simulink model "GridConnected200921_DSMC_OK_2018"  (R2022b)
settings: Solver=ode45  StartTime=0.0  StopTime=1  RelTol=1e-3
InitFcn:
  | %tham so mach nghich luu nguon ap mot pha
  | Li = 0.423e-3+0.429e-3;
  | rLi = 0.172+0.167;
  | Lg = 0.795e-3;
  | rLg = 0.36;
  | 
  | Lf = 0.8*(Li+Lg);
  | rL = (rLi+rLg);
  | 
  | Cdc = 0.9*2*470e-6;
  | P = 2500;  %Cong suat 2.5kW
  | VdcRated = 400; %Dien ap dat 400VDC
  | Rmin = (VdcRated^2)/P; %Full load
  | Rmax = (VdcRated^2)/(0.05*P); % 5% load
  | Fs = 10000;
  | Ts = 1/Fs;
StopFcn:
  | figure(1);
  | subplot(2,1,1); hold on; grid on;
  | plot(Vdc_Ref.time, Vdc_Ref.signals.values,'-k','Linewidth',1.5);
  | plot(Vdc_Fb.time, Vdc_Fb.signals.values,'r','Linewidth',1.5);
  | plot(Vdc_Filter.time, Vdc_Filter.signals.values,'b','Linewidth',1.5);
  | legend('Vdc Ref','Vdc Fb','Vdc Filter');
  | xlabel('Time(s)'); ylabel('Dc bus voltage(V)');
  | 
  | subplot(2,1,2); hold on; grid on;
  | [hAx,hLine1,hLine2] = plotyy(P.time, P.signals.values./1000, Q.time, Q.signals.values./1000);
  | set(hAx(1),'YLim',[-10 10]);
  | set(hAx(2),'YLim',[-10 10]);
  | set(hAx(1),'YTick',[-10:5:10]);
  | set(hAx(2),'YTick',[-10:5:10]);
  | ylabel(hAx(1),'P(kW)'); ylabel(hAx(2),'Q(kVar)');
  | legend('Active power','Reactive power');
  | set(hAx(1),'Fontsize',20);
  | set(hAx(2),'Fontsize',20)
  | xlabel('Time(s)'); ylabel('Injected power');
  | 
  | figure(2);
  | hold on; grid on;
  | plot(iL_Ref.time, iL_Ref.signals.values,'-.g','Linewidth',1.5);
  | plot(iL_avg.time, iL_avg.signals.values,'r','Linewidth',1.5);
  | plot(iL.time, iL.signals.values,'b','Linewidth',1.5);
  | legend('iL Ref','iL average','iL');
  | xlabel('Time(s)'); ylabel('Output current(A)');
  | %magnifyOnFigure();
  | 
  | figure(3);
  | subplot(2,1,1); hold on; grid on;
  | [hAx,hLine1,hLine2] = plotyy(V_Line.time, V_Line.signals.values, iL.time, iL.signals.values);
  | set(hAx(1),'YLim',[-400 400]);
  | set(hAx(2),'YLim',[-60 60]);
  | set(hAx(1),'YTick',[-400:200:400]);
  | set(hAx(2),'YTick',[-60:30:60]);
  | ylabel(hAx(1),'Line voltage(V)'); ylabel(hAx(2),'Injected current(A)');
  | legend('Line voltage','Injected current');
  | set(hAx(1),'Fontsize',20);
  | set(hAx(2),'Fontsize',20)
  | xlabel('Time(s)');
  | 
  | subplot(2,1,2);  hold on; grid on;
  | plot(Vdc_Ref.time, Vdc_Ref.signals.values,'-k','Linewidth',1.5);
  | plot(Vdc_Fb.time, Vdc_Fb.signals.values,'r','Linewidth',1.5);
  | plot(Vdc_Filter.time, Vdc_Filter.signals.values,'b','Linewidth',1.5);
  | legend('Vdc Ref','Vdc Fb','Vdc Filter');
  | xlabel('Time(s)'); ylabel('Dc bus voltage(V)');
  | %magnifyOnFigure();
  | 
  | figure(4);
  | subplot(2,1,1); hold on; grid on;
  | plot(V_Line.time, V_Line.signals.values,'r','Linewidth',1.5);
  | subplot(2,1,2); hold on; grid on;
  | plot(Theta.time, Theta.signals.values,'b','Linewidth',1.5);
  | 
  | figure(5);
  | subplot(2,1,1); hold on; grid on;
  | plot(V_Line.time, V_Line.signals.values,'r','Linewidth',1.5);
  | xlabel('Time(s)'); ylabel('Line voltage(V)');
  | subplot(2,1,2); hold on; grid on;
  | plot(iL.time, iL.signals.values,'b','Linewidth',1.5);
  | xlabel('Time(s)'); ylabel('Injected current(A)');
undefined symbols (not defined in the file): Vdc
libraries: spsSeriesRLCBranchLib x7, spsVoltageMeasurementLib x5, spsIGBTLib x4, spsIGBTDiodeLib x4, spsBreakerLib x3, spsCurrentMeasurementLib x2, spsControlledVoltageSourceLib x1, spsControlledCurrentSourceLib x1, spsTriangleGeneratorLib x1, spspowerguiLib x1
settings Model: Creator=ADMIN  LastModifiedBy=Dell
settings SolverCC: AlgebraicLoopSolver=TrustRegion
settings DataIOCC: ReturnWorkspaceOutputs=off
settings DebuggingCC: UnconnectedInputMsg=warning  UnconnectedOutputMsg=warning  UnconnectedLineMsg=warning  SFMachineParentedDataDiag=warning  ArithmeticOperatorsInVariantConditions=warning
settings ModelReferenceCC: EnableRefExpFcnMdlSchedulingChecks=on
settings SFSimCC: SimUseLocalCustomCode=off  CustomCodeUndefinedFunction=UseInterfaceOnly
settings RTWCC: RTWUseLocalCustomCode=off

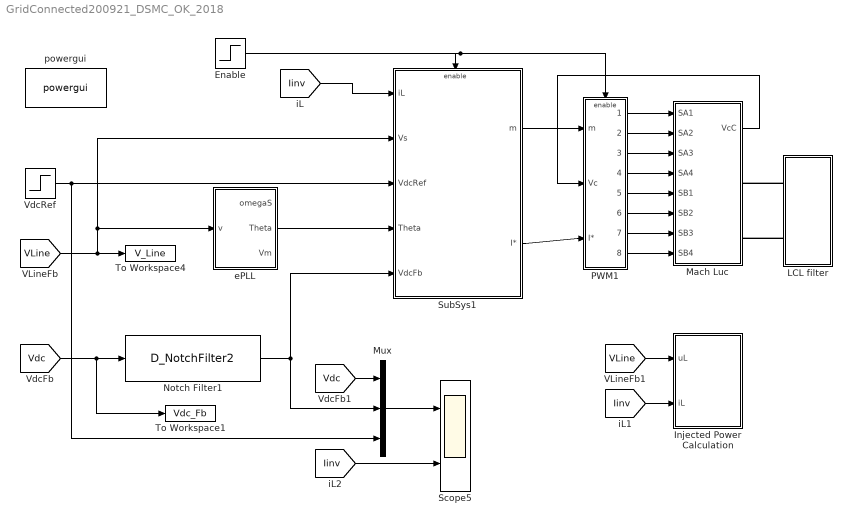
== system GridConnected200921_DSMC_OK_2018 ==
  Enable : Step  Time=0.1  SampleTime=0
  Injected Power Calculation : Subsystem
  LCL filter : Subsystem
  Mach Luc : Subsystem
  Mux : Mux  Inputs=3
  Notch Filter1 : S-Function  InitFcn=try, set_param(gcb,'FunctionName','D_NotchFilter2'), end  FunctionName=D_NotchFilter2  SFunctionModules=D_NotchFilter2_wrapper  SFunctionDeploymentMode=off  EnableBusSupport=off  mask(S-Function Builder){}
      mask help: Simulink:masks:SFunctionBuilder_MD
      mask init:
      | val = [[.9  0.75 0.75 1 1 .9 .9 1]',[1 1 0.75 0.75 .9 .9 1 .9]'];try , sys = get_param(gcb,'SfunBuilderFcnName');if isempty(sys), sys = get_param(gcb,'FunctionName'); end,catch, sys = get_param(gcb,'FunctionName'); end
      settings: CopyFcn=set_param(gcbh,'LinkStatus','none')  PreSaveFcn=try, set_param(gcb,'FunctionName','D_NotchFilter2'), end  OpenFcn=sfunctionwizard(gcbh)
      mask Display: plot(val(:,1),val(:,2)),disp(sys), port_label('input',1,'uDC'), port_label('output',1,'uDCav')
  PWM1 : Subsystem
  Scope5 : Scope  NumInputPorts=2
  SubSys1 : Subsystem
  To Workspace1 : ToWorkspace  VariableName=Vdc_Fb  SaveFormat=Structure With Time  SampleTime=1e-4
  To Workspace4 : ToWorkspace  VariableName=V_Line  SaveFormat=Structure With Time  SampleTime=1e-4
  VdcRef : Step  Time=0  After=400  SampleTime=0
  ePLL : Subsystem
  powergui : spspowerguiLib/powergui  Priority=1  SimulationMode=Discrete  SampleTime=5e-8  frequency=60  Iterations=50  frequencyindice=0  Pbase=100e6  ErrMax=1e-4  UnitsV=kV  UnitsW=MW  buscounter=0  FunctionMessages=off  echomessages=off  EnableUseOfTLC=off  CurrentSourceSwitches=off  DisableSnubberDevices=off  DisableRonSwitches=off  DisableVfSwitches=off  DisplayEquations=off  AutomaticDiscreteSolvers=off  SolverType=Tustin/Backward Euler (TBE)  Interpol=off  ExternalGateDelay=off  methode=off  Ts=100  x0status=blocks  SPID=off  SwTol=0  HookPort=off  NonlinearTolerance=1e-4  nMaxIteration=100  ContinueOnMaxIteration=off  RestoreLinks=warning  ResistiveCurrentMeasurement=off  Frange=[0:2:500]  Ylog=off  Xlog=on  ShowGrid=off  save=off  variable=ZData  structure=iL  ZoomFFT=on  StartTime=0.5  cycles=4  DisplayStyle=2  fundamental=50  FreqAxis=off  MaxFrequency=10000  frequencyindicesteady=1  RmsSteady=1  display=off
  wires:
  VdcRef/1 -> Mux/3, SubSys1/3(VdcRef)
  [VLine] -> SubSys1/2(Vs), ePLL/1(v), To Workspace4/1
  ePLL/2(Theta) -> SubSys1/4(Theta)
  Enable/1 -> SubSys1/Enable, PWM1/Enable
  [Iinv] -> SubSys1/1(iL)
  SubSys1/1(m) -> PWM1/1(m)
  PWM1/8(SB4) -> Mach Luc/8(SB4)
  PWM1/7(SB3) -> Mach Luc/7(SB3)
  PWM1/6(SB2) -> Mach Luc/6(SB2)
  PWM1/5(SB1) -> Mach Luc/5(SB1)
  PWM1/4(SA4) -> Mach Luc/4(SA4)
  PWM1/3(SA3) -> Mach Luc/3(SA3)
  PWM1/2(SA2) -> Mach Luc/2(SA2)
  PWM1/1(SA1) -> Mach Luc/1(SA1)
  Mach Luc/1(VcC) -> PWM1/2(Vc)
  SubSys1/2(I*) -> PWM1/3(I*)
  [Iinv] -> Injected Power Calculation/2(iL)
  [VLine] -> Injected Power Calculation/1(uL)
  Mux/1 -> Scope5/1
  [Vdc] -> Notch Filter1/1, To Workspace1/1
  Notch Filter1/1 -> Mux/2, SubSys1/5(VdcFb)
  [Vdc] -> Mux/1
  [Iinv] -> Scope5/2
  connections:
  LCL filter/LConn1 -- Mach Luc/RConn1
  LCL filter/LConn2 -- Mach Luc/RConn2

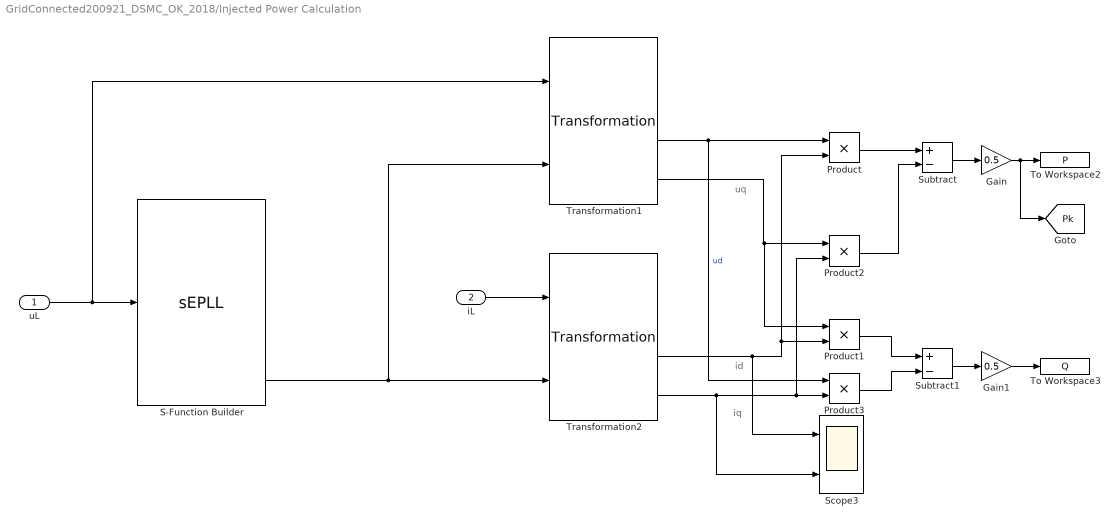
== system GridConnected200921_DSMC_OK_2018/Injected Power Calculation ==
  note: uq
  note: id
  note: iq
  uL : Inport
  iL : Inport  Port=2
  Gain : Gain  Gain=0.5
  Gain1 : Gain  Gain=0.5
  Product{,1..3} (4 alike) : Product
  S-Function Builder : S-Function  InitFcn=try, set_param(gcb,'FunctionName','sEPLL'), end  FunctionName=sEPLL  SFunctionModules=sEPLL_wrapper  SFunctionDeploymentMode=off  EnableBusSupport=off  mask(S-Function Builder){}
      mask help: Simulink:masks:SFunctionBuilder_MD
      mask init: same as GridConnected200921_DSMC_OK_2018/Notch Filter1
      settings: CopyFcn=set_param(gcbh,'LinkStatus','none')  PreSaveFcn=try, set_param(gcb,'FunctionName','sEPLL'), end  OpenFcn=sfunctionwizard(gcbh)
      mask Display: plot(val(:,1),val(:,2)),disp(sys), port_label('input',1,'uk'), port_label('output',1,'Ak1'), port_label('output',2,'Phik1'), port_label('output',3,'Omegak1'), port_label('output',4,'SinPhi'), port_label('output',5,'Phik_90Shift')
  Scope3 : Scope  NumInputPorts=2
  Subtract : Sum  Inputs=+-
  Subtract1 : Sum  Inputs=+-
  To Workspace2 : ToWorkspace  VariableName=P  SaveFormat=Structure With Time  SampleTime=1e-4
  To Workspace3 : ToWorkspace  VariableName=Q  SaveFormat=Structure With Time  SampleTime=1e-4
  Transformation1 : S-Function  InitFcn=try, set_param(gcb,'FunctionName','Transformation'), end  FunctionName=Transformation  SFunctionModules=Transformation_wrapper  SFunctionDeploymentMode=off  EnableBusSupport=off  mask(S-Function Builder){}
      mask help: Simulink:masks:SFunctionBuilder_MD
      mask init: same as GridConnected200921_DSMC_OK_2018/Notch Filter1
      settings: CopyFcn=set_param(gcbh,'LinkStatus','none')  PreSaveFcn=try, set_param(gcb,'FunctionName','Transformation'), end  OpenFcn=sfunctionwizard(gcbh)
      mask Display: plot(val(:,1),val(:,2)),disp(sys), port_label('input',1,'u'), port_label('input',2,'Theta'), port_label('output',1,'yAlpha'), port_label('output',2,'yBeta'), port_label('output',3,'yD'), port_label('output',4,'yQ')
  Transformation2 : S-Function  InitFcn=try, set_param(gcb,'FunctionName','Transformation'), end  FunctionName=Transformation  SFunctionModules=Transformation_wrapper  SFunctionDeploymentMode=off  EnableBusSupport=off  mask(S-Function Builder){}
      mask help: Simulink:masks:SFunctionBuilder_MD
      mask init: same as GridConnected200921_DSMC_OK_2018/Notch Filter1
      settings: CopyFcn=set_param(gcbh,'LinkStatus','none')  PreSaveFcn=try, set_param(gcb,'FunctionName','Transformation'), end  OpenFcn=sfunctionwizard(gcbh)
      mask Display: plot(val(:,1),val(:,2)),disp(sys), port_label('input',1,'u'), port_label('input',2,'Theta'), port_label('output',1,'yAlpha'), port_label('output',2,'yBeta'), port_label('output',3,'yD'), port_label('output',4,'yQ')
  tag scope: Pk=global
  wires:
  uL/1 -> Transformation1/1, S-Function Builder/1
  S-Function Builder/5 -> Transformation2/2, Transformation1/2
  iL/1 -> Transformation2/1
  Transformation1/3 -> Product3/1, Product/1  "ud"
  Transformation1/4 -> Product1/1, Product2/1
  Transformation2/3 -> Scope3/1, Product1/2, Product/2
  Transformation2/4 -> Scope3/2, Product3/2, Product2/2
  Product/1 -> Subtract/1
  Product2/1 -> Subtract/2
  Subtract/1 -> Gain/1
  Product1/1 -> Subtract1/1
  Product3/1 -> Subtract1/2
  Subtract1/1 -> Gain1/1
  Gain/1 -> [Pk], To Workspace2/1
  Gain1/1 -> To Workspace3/1

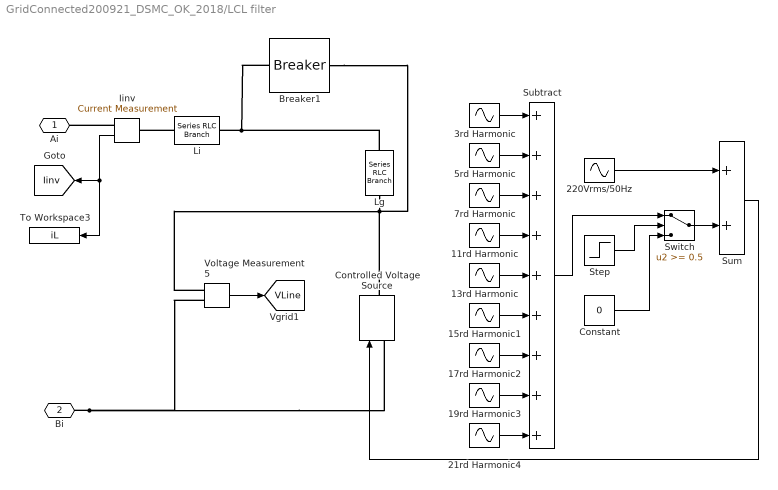
== system GridConnected200921_DSMC_OK_2018/LCL filter ==
  "11rd Harmonic " : Sin  Amplitude=220*sqrt(2)*0.04  Frequency=2*pi*50*11  SampleTime=0
  13rd Harmonic : Sin  Amplitude=220*sqrt(2)*0.12  Frequency=2*pi*50*13  SampleTime=0
  15rd Harmonic1 : Sin  Amplitude=220*sqrt(2)*0.01  Frequency=2*pi*50*15  SampleTime=0
  17rd Harmonic2 : Sin  Amplitude=220*sqrt(2)*0.07  Frequency=2*pi*50*17  SampleTime=0
  19rd Harmonic3 : Sin  Amplitude=220*sqrt(2)*0.09  Frequency=2*pi*50*19  SampleTime=0
  21rd Harmonic4 : Sin  Amplitude=220*sqrt(2)*0.018  Frequency=2*pi*50*21  SampleTime=0
  220Vrms/50Hz : Sin  Amplitude=220*sqrt(2)  Frequency=2*pi*50  SampleTime=0
  3rd Harmonic : Sin  Amplitude=220*sqrt(2)*0.1  Frequency=2*pi*50*3  SampleTime=0
  5rd Harmonic : Sin  Amplitude=220*sqrt(2)*0.05  Frequency=2*pi*50*5  SampleTime=0
  7rd Harmonic : Sin  Amplitude=220*sqrt(2)*0.02  Frequency=2*pi*50*7  SampleTime=0
  Breaker1 : spsBreakerLib/Breaker  InitialState=0  SwitchingTimes=0.7  External=off  BreakerResistance=0.001  SnubberResistance=1e6  SnubberCapacitance=inf  Measurements=None  MoreParameters=on  NoBreakLoop=off
  Constant : Constant  Value=0
  Controlled Voltage Source : spsControlledVoltageSourceLib/Controlled Voltage Source  Initialize=on  Source_Type=AC  Amplitude=0  Phase=0  Frequency=0  Measurements=None
  Iinv : spsCurrentMeasurementLib/Current Measurement  PhasorSimulation=off  OutputType=Complex  PSBequivalent=0
  Lg : spsSeriesRLCBranchLib/Series RLC Branch  LConnTagsString=__new0  RConnTagsString=__new0  BranchType=RL  Resistance=rLg  Inductance=Lg*1.0  SetiL0=off  InitialCurrent=0  Capacitance=1e-6  Setx0=off  InitialVoltage=0  Measurements=None
  Li : spsSeriesRLCBranchLib/Series RLC Branch  LConnTagsString=__new0  RConnTagsString=__new0  BranchType=RL  Resistance=rLi  Inductance=Li*1.0  SetiL0=off  InitialCurrent=0  Capacitance=1e-6  Setx0=off  InitialVoltage=0  Measurements=None
  Step : Step  Time=0.75  SampleTime=0
  Subtract : Sum  Inputs=+++++++++
  Sum : Sum  InputSameDT=on  SaturateOnIntegerOverflow=on  OutDataTypeStr=Inherit: Same as first input
  Switch : Switch  Threshold=0.5
  To Workspace3 : ToWorkspace  VariableName=iL  SaveFormat=Structure With Time  SampleTime=5e-8
  Voltage Measurement5 : spsVoltageMeasurementLib/Voltage Measurement  PhasorSimulation=off  OutputType=Complex  PSBequivalent=0
  Ai : PMIOPort  Side=Left
  Bi : PMIOPort  Port=2  Side=Left
  tag scope: Iinv=global, VLine=global
  wires:
  Voltage Measurement5/1 -> [VLine]
  Iinv/1 -> To Workspace3/1, [Iinv]
  Switch/1 -> Sum/2
  Constant/1 -> Switch/3
  Step/1 -> Switch/2
  220Vrms/50Hz/1 -> Sum/1
  7rd Harmonic/1 -> Subtract/3
  5rd Harmonic/1 -> Subtract/2
  3rd Harmonic/1 -> Subtract/1
  "11rd Harmonic "/1 -> Subtract/4
  13rd Harmonic/1 -> Subtract/5
  Subtract/1 -> Switch/1
  Sum/1 -> Controlled Voltage Source/1
  21rd Harmonic4/1 -> Subtract/9
  19rd Harmonic3/1 -> Subtract/8
  17rd Harmonic2/1 -> Subtract/7
  15rd Harmonic1/1 -> Subtract/6
  connections:
  Bi/RConn1 -- Voltage Measurement5/LConn2 -- Controlled Voltage Source/LConn1
  Li/LConn1 -- Iinv/LConn1
  Iinv/RConn1 -- Ai/RConn1
  Lg/RConn1 -- Breaker1/RConn1 -- Controlled Voltage Source/RConn1 -- Voltage Measurement5/LConn1
  Breaker1/LConn1 -- Lg/LConn1 -- Li/RConn1

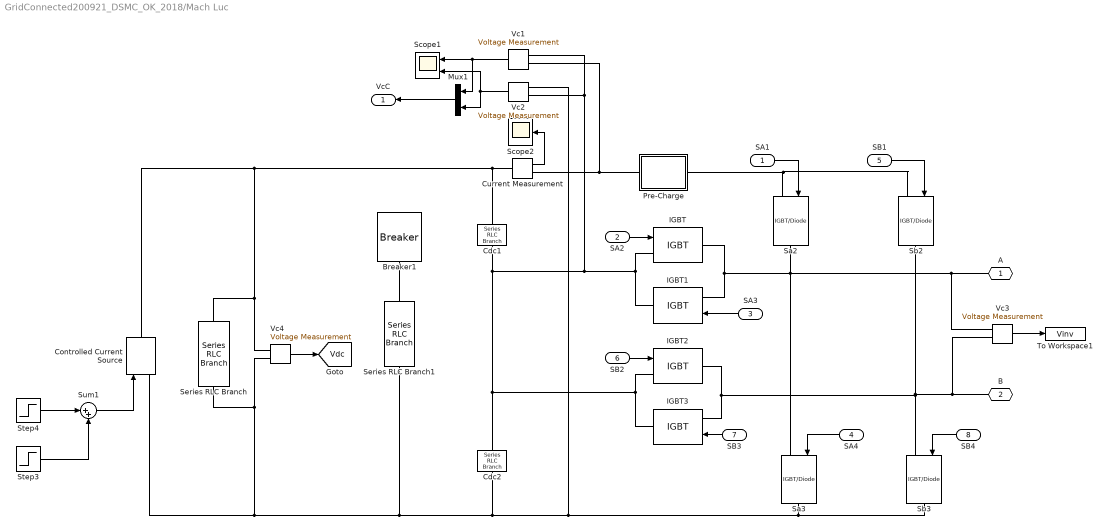
== system GridConnected200921_DSMC_OK_2018/Mach Luc ==
  SA1 : Inport
  SA2 : Inport  Port=2
  SA3 : Inport  Port=3
  SA4 : Inport  Port=4
  SB1 : Inport  Port=5
  SB2 : Inport  Port=6
  SB3 : Inport  Port=7
  SB4 : Inport  Port=8
  Breaker1 : spsBreakerLib/Breaker  InitialState=0  SwitchingTimes=0.1  External=off  BreakerResistance=0.001  SnubberResistance=1e6  SnubberCapacitance=inf  Measurements=None  MoreParameters=on  NoBreakLoop=off
  Cdc1 : spsSeriesRLCBranchLib/Series RLC Branch  LConnTagsString=__new0  RConnTagsString=__new0  BranchType=RC  Resistance=0.01  Inductance=0  SetiL0=off  InitialCurrent=0  Capacitance=940e-6  Setx0=off  InitialVoltage=Vdc/2-100  Measurements=Branch voltage and current
  Cdc2 : spsSeriesRLCBranchLib/Series RLC Branch  LConnTagsString=__new0  RConnTagsString=__new0  BranchType=RC  Resistance=0.01  Inductance=0  SetiL0=off  InitialCurrent=0  Capacitance=940e-6  Setx0=off  InitialVoltage=Vdc/2+100  Measurements=Branch voltage and current
  Controlled Current Source : spsControlledCurrentSourceLib/Controlled Current Source  Initialize=on  Source_Type=DC  Amplitude=0  Phase=0  Frequency=0  Measurements=None
  Current Measurement : spsCurrentMeasurementLib/Current Measurement  PhasorSimulation=off  OutputType=Complex  PSBequivalent=0
  IGBT{,1..3} (4 alike) : spsIGBTLib/IGBT  Ron=0.001  Lon=0  Vf=1  Tf=1e-6  Tt=2e-6  IC=0  Rs=1e5  Cs=inf  Measurements=off
  Mux1 : Mux  Inputs=2
  Pre-Charge : Subsystem
  Sa2 : spsIGBTDiodeLib/IGBT//Diode  Ron=1e-3  Rs=1e5  Cs=inf  Measurements=off
  Sa3 : spsIGBTDiodeLib/IGBT//Diode  Ron=1e-3  Rs=1e5  Cs=inf  Measurements=off
  Sb2 : spsIGBTDiodeLib/IGBT//Diode  Ron=1e-3  Rs=1e5  Cs=inf  Measurements=off
  Sb3 : spsIGBTDiodeLib/IGBT//Diode  Ron=1e-3  Rs=1e5  Cs=inf  Measurements=off
  Scope1 : Scope  NumInputPorts=2
  Scope2 : Scope
  Series RLC Branch : spsSeriesRLCBranchLib/Series RLC Branch  LConnTagsString=__new0  RConnTagsString=__new0  BranchType=RC  Resistance=0.1  Inductance=1e-3  SetiL0=off  InitialCurrent=0  Capacitance=Cdc  Setx0=off  InitialVoltage=0  Measurements=None
  Series RLC Branch1 : spsSeriesRLCBranchLib/Series RLC Branch  LConnTagsString=__new0  RConnTagsString=__new0  BranchType=R  Resistance=400*400/100  Inductance=1e-3  SetiL0=off  InitialCurrent=0  Capacitance=Cdc  Setx0=off  InitialVoltage=0  Measurements=None
  Step3 : Step  Time=0.5  After=20  SampleTime=0
  Step4 : Step  Time=0.15  After=-10  SampleTime=0
  Sum1 : Sum  Inputs=|++
  To Workspace1 : ToWorkspace  VariableName=Vinv  SaveFormat=Structure With Time  SampleTime=1e-4
  Vc{1..4} (4 alike) : spsVoltageMeasurementLib/Voltage Measurement  PhasorSimulation=off  OutputType=Complex  PSBequivalent=0
  A : PMIOPort  Side=Right
  B : PMIOPort  Port=2  Side=Right
  VcC : Outport  VectorParamsAs1DForOutWhenUnconnected=off
  tag scope: Vdc=global
  wires:
  Vc4/1 -> [Vdc]
  Vc2/1 -> Mux1/2, Scope1/2
  Vc1/1 -> Mux1/1, Scope1/1
  SB3/1 -> IGBT3/1
  SA2/1 -> IGBT/1
  Mux1/1 -> VcC/1
  SB2/1 -> IGBT2/1
  SA4/1 -> Sa3/1
  SB4/1 -> Sb3/1
  SB1/1 -> Sb2/1
  SA1/1 -> Sa2/1
  SA3/1 -> IGBT1/1
  Sum1/1 -> Controlled Current Source/1
  Step4/1 -> Sum1/1
  Step3/1 -> Sum1/2
  Vc3/1 -> To Workspace1/1
  Current Measurement/1 -> Scope2/1
  connections:
  Sb3/RConn1 -- Series RLC Branch1/RConn1 -- Series RLC Branch/RConn1 -- Vc4/LConn2 -- Controlled Current Source/LConn1 -- Cdc2/RConn1 -- Vc2/LConn2 -- Sa3/RConn1
  IGBT/LConn1 -- IGBT1/RConn1 -- Vc1/LConn2 -- Vc2/LConn1 -- Cdc1/RConn1 -- IGBT2/LConn1 -- IGBT3/RConn1 -- Cdc2/LConn1
  Vc4/LConn1 -- Series RLC Branch/LConn1 -- Cdc1/LConn1 -- Current Measurement/LConn1 -- Controlled Current Source/RConn1
  IGBT2/RConn1 -- Vc3/LConn2 -- B/RConn1 -- Sb2/RConn1 -- Sb3/LConn1 -- IGBT3/LConn1
  IGBT/RConn1 -- Vc3/LConn1 -- A/RConn1 -- Sa3/LConn1 -- Sa2/RConn1 -- IGBT1/LConn1
  Pre-Charge/RConn1 -- Sb2/LConn1 -- Sa2/LConn1
  Vc1/LConn1 -- Current Measurement/RConn1 -- Pre-Charge/LConn1
  Breaker1/RConn1 -- Series RLC Branch1/LConn1

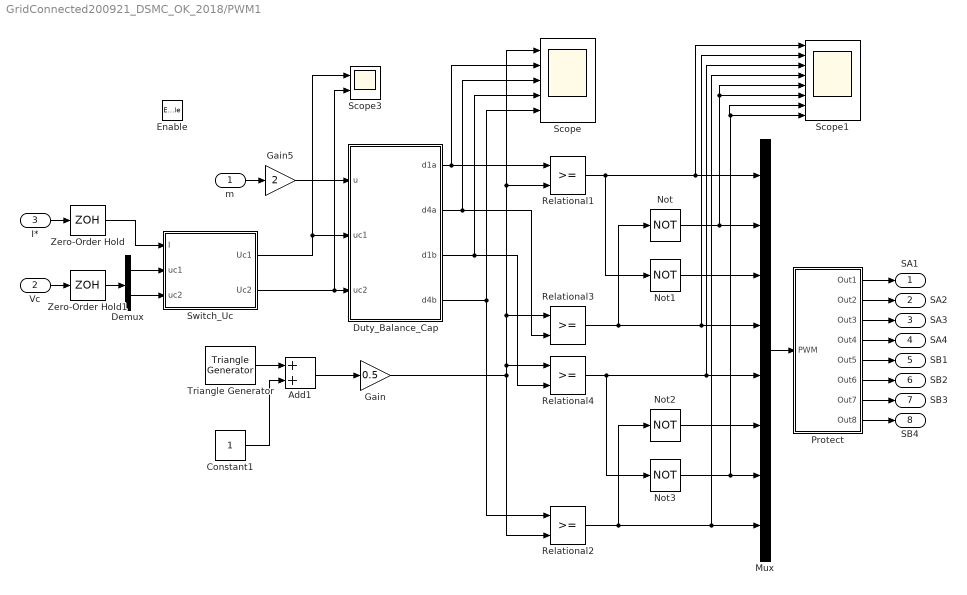
== system GridConnected200921_DSMC_OK_2018/PWM1 ==
  m : Inport
  Vc : Inport  Port=2
  I* : Inport  Port=3
  Enable : EnablePort
  Add1 : Sum
  Constant1 : Constant
  Demux : Demux  Outputs=2
  Duty_Balance_Cap : MATLAB Function  TreatAsAtomicUnit=on
  Gain : Gain  Gain=0.5
  Gain5 : Gain  Gain=2
  Mux : Mux  Inputs=8
  Not{,1..3} (4 alike) : Logic  Operator=NOT  AllPortsSameDT=off  OutDataTypeStr=boolean
  Protect : Subsystem
  Relational{1..4} (4 alike) : RelationalOperator  OutDataTypeStr=boolean
  Scope : Scope  NumInputPorts=5
  Scope1 : Scope  NumInputPorts=8
  Scope3 : Scope  NumInputPorts=2
  Switch_Uc : MATLAB Function  TreatAsAtomicUnit=on
  Triangle Generator : spsTriangleGeneratorLib/Triangle Generator  Freq=10000  Phase=0  Ts=0
  Zero-Order Hold : ZeroOrderHold  SampleTime=1/5000
  Zero-Order Hold1 : ZeroOrderHold  SampleTime=1/5000
  SA1 : Outport  VectorParamsAs1DForOutWhenUnconnected=off
  SA2 : Outport  Port=2  VectorParamsAs1DForOutWhenUnconnected=off
  SA3 : Outport  Port=3  VectorParamsAs1DForOutWhenUnconnected=off
  SA4 : Outport  Port=4  VectorParamsAs1DForOutWhenUnconnected=off
  SB1 : Outport  Port=5  VectorParamsAs1DForOutWhenUnconnected=off
  SB2 : Outport  Port=6  VectorParamsAs1DForOutWhenUnconnected=off
  SB3 : Outport  Port=7  VectorParamsAs1DForOutWhenUnconnected=off
  SB4 : Outport  Port=8  VectorParamsAs1DForOutWhenUnconnected=off
  wires:
  Add1/1 -> Gain/1
  Constant1/1 -> Add1/2
  Gain/1 -> Relational4/1, Relational1/2, Scope/1, Relational3/1, Relational2/2
  m/1 -> Gain5/1
  Gain5/1 -> Duty_Balance_Cap/1(u)
  Duty_Balance_Cap/1(d1a) -> Relational1/1, Scope/2
  Duty_Balance_Cap/2(d4a) -> Scope/3, Relational3/2
  Duty_Balance_Cap/3(d1b) -> Relational4/2, Scope/4
  Duty_Balance_Cap/4(d4b) -> Relational2/1, Scope/5
  Switch_Uc/1(Uc1) -> Duty_Balance_Cap/2(uc1), Scope3/1
  Switch_Uc/2(Uc2) -> Duty_Balance_Cap/3(uc2), Scope3/2
  Relational1/1 -> Scope1/1, Mux/1, Not1/1
  Not/1 -> Scope1/6, Scope1/5, Mux/2
  Relational3/1 -> Scope1/2, Mux/4, Not/1
  Relational4/1 -> Scope1/3, Mux/5, Not3/1
  Not3/1 -> Scope1/8, Scope1/7, Mux/7
  Relational2/1 -> Scope1/4, Mux/8, Not2/1
  Triangle Generator/1 -> Add1/1
  Mux/1 -> Protect/1(PWM)
  Protect/1(Out1) -> SA1/1
  Protect/2(Out2) -> SA2/1
  Protect/3(Out3) -> SA3/1
  Protect/4(Out4) -> SA4/1
  Protect/5(Out5) -> SB1/1
  Protect/6(Out6) -> SB2/1
  Protect/7(Out7) -> SB3/1
  Protect/8(Out8) -> SB4/1
  Not1/1 -> Mux/3
  Not2/1 -> Mux/6
  Vc/1 -> Zero-Order Hold1/1
  Zero-Order Hold1/1 -> Demux/1
  Demux/1 -> Switch_Uc/2(uc1)
  Demux/2 -> Switch_Uc/3(uc2)
  Zero-Order Hold/1 -> Switch_Uc/1(I)
  I*/1 -> Zero-Order Hold/1

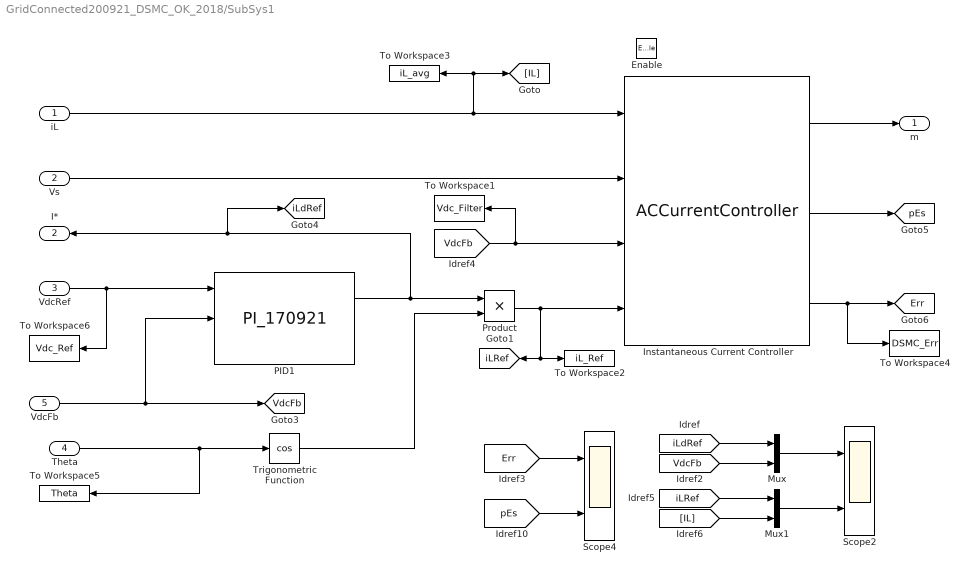
== system GridConnected200921_DSMC_OK_2018/SubSys1 ==
  iL : Inport
  Vs : Inport  Port=2
  VdcRef : Inport  Port=3
  Theta : Inport  Port=4
  VdcFb : Inport  Port=5
  Enable : EnablePort
  Instantaneous Current Controller : S-Function  InitFcn=try, set_param(gcb,'FunctionName','ACCurrentController'), end  FunctionName=ACCurrentController  SFunctionModules=ACCurrentController_wrapper  SFunctionDeploymentMode=off  EnableBusSupport=off  mask(S-Function Builder){}
      mask help: Simulink:masks:SFunctionBuilder_MD
      mask init: same as GridConnected200921_DSMC_OK_2018/Notch Filter1
      settings: CopyFcn=set_param(gcbh,'LinkStatus','none')  PreSaveFcn=try, set_param(gcb,'FunctionName','ACCurrentController'), end  OpenFcn=sfunctionwizard(gcbh)
      mask Display: plot(val(:,1),val(:,2)),disp(sys), port_label('input',1,'iLk'), port_label('input',2,'vLk'), port_label('input',3,'Vdck'), port_label('input',4,'iLkRef'), port_label('output',1,'mk'), port_label('output',2,'Pk'), port_label('output',3,'error')
  Mux : Mux  Inputs=2
  Mux1 : Mux  Inputs=2
  PID1 : S-Function  InitFcn=try, set_param(gcb,'FunctionName','PI_170921'), end  FunctionName=PI_170921  SFunctionModules=PI_170921_wrapper  SFunctionDeploymentMode=off  EnableBusSupport=off  mask(S-Function Builder){}
      mask help: Simulink:masks:SFunctionBuilder_MD
      mask init: same as GridConnected200921_DSMC_OK_2018/Notch Filter1
      settings: CopyFcn=set_param(gcbh,'LinkStatus','none')  PreSaveFcn=try, set_param(gcb,'FunctionName','PI_170921'), end  OpenFcn=sfunctionwizard(gcbh)
      mask Display: plot(val(:,1),val(:,2)),disp(sys), port_label('input',1,'VdcRef'), port_label('input',2,'VdcFb'), port_label('input',3,'Pes'), port_label('output',1,'usk'), port_label('output',2,'uD')
  Product : Product
  Scope2 : Scope  NumInputPorts=2
  Scope4 : Scope  NumInputPorts=2
  To Workspace1 : ToWorkspace  VariableName=Vdc_Filter  SaveFormat=Structure With Time  SampleTime=0.0025
  To Workspace2 : ToWorkspace  VariableName=iL_Ref  SaveFormat=Structure With Time  SampleTime=1e-4
  To Workspace3 : ToWorkspace  VariableName=iL_avg  SaveFormat=Structure With Time  SampleTime=1e-4
  To Workspace4 : ToWorkspace  VariableName=DSMC_Err  SaveFormat=Structure With Time  SampleTime=0.0025
  To Workspace5 : ToWorkspace  VariableName=Theta  SaveFormat=Structure With Time  SampleTime=1e-4
  To Workspace6 : ToWorkspace  VariableName=Vdc_Ref  SaveFormat=Structure With Time  SampleTime=0.0025
  Trigonometric Function : Trigonometry  Operator=cos
  m : Outport  VectorParamsAs1DForOutWhenUnconnected=off
  I* : Outport  Port=2  VectorParamsAs1DForOutWhenUnconnected=off
  tag scope: Err=global, VdcFb=global, iLRef=global, iLdRef=global, pEs=global
  wires:
  VdcRef/1 -> PID1/1, To Workspace6/1
  Vs/1 -> Instantaneous Current Controller/2
  VdcFb/1 -> PID1/2, [VdcFb]
  Trigonometric Function/1 -> Product/2
  Product/1 -> Instantaneous Current Controller/4, To Workspace2/1, [iLRef]
  Theta/1 -> Trigonometric Function/1, To Workspace5/1
  [VdcFb] -> Instantaneous Current Controller/3, To Workspace1/1
  iL/1 -> Instantaneous Current Controller/1, To Workspace3/1, [IL]
  PID1/1 -> [iLdRef], I*/1, Product/1
  [iLdRef] -> Mux/1
  Mux/1 -> Scope2/1
  [iLRef] -> Mux1/1
  [IL] -> Mux1/2
  Mux1/1 -> Scope2/2
  [VdcFb] -> Mux/2
  [Err] -> Scope4/1
  [pEs] -> Scope4/2
  Instantaneous Current Controller/1 -> m/1
  Instantaneous Current Controller/2 -> [pEs]
  Instantaneous Current Controller/3 -> To Workspace4/1, [Err]

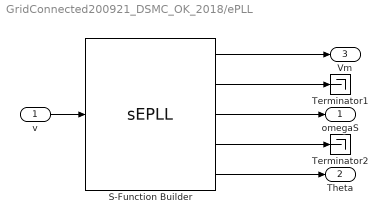
== system GridConnected200921_DSMC_OK_2018/ePLL ==
  v : Inport
  S-Function Builder : S-Function  InitFcn=try, set_param(gcb,'FunctionName','sEPLL'), end  FunctionName=sEPLL  SFunctionModules=sEPLL_wrapper.c  SFunctionDeploymentMode=off  EnableBusSupport=off  mask(S-Function Builder){}
      mask help: Simulink:masks:SFunctionBuilder_MD
      mask init: same as GridConnected200921_DSMC_OK_2018/Notch Filter1
      settings: CopyFcn=set_param(gcbh,'LinkStatus','none')  PreSaveFcn=try, set_param(gcb,'FunctionName','sEPLL'), end  OpenFcn=sfunctionwizard(gcbh)
      mask Display:
      | plot(val(:,1),val(:,2))
      | disp(sys)
      | port_label('input',1,'uk')
      | port_label('output',1,'Ak1')
      | port_label('output',2,'Phik1')
      | port_label('output',3,'Omegak1')
      | port_label('output',4,'SinPhi')
      | port_label('output',5,'Phik_90Shift')
  Terminator1 : Terminator
  Terminator2 : Terminator
  omegaS : Outport  VectorParamsAs1DForOutWhenUnconnected=off
  Theta : Outport  Port=2  VectorParamsAs1DForOutWhenUnconnected=off
  Vm : Outport  Port=3  VectorParamsAs1DForOutWhenUnconnected=off
  wires:
  v/1 -> S-Function Builder/1
  S-Function Builder/4 -> Terminator2/1
  S-Function Builder/1 -> Vm/1
  S-Function Builder/2 -> Terminator1/1
  S-Function Builder/3 -> omegaS/1
  S-Function Builder/5 -> Theta/1

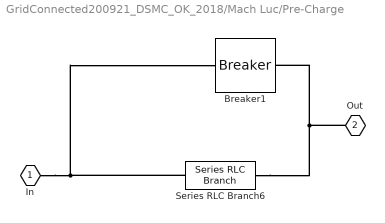
== system GridConnected200921_DSMC_OK_2018/Mach Luc/Pre-Charge ==
  Breaker1 : spsBreakerLib/Breaker  InitialState=0  SwitchingTimes=0.04  External=off  BreakerResistance=0.001  SnubberResistance=1e6  SnubberCapacitance=inf  Measurements=None  MoreParameters=on  NoBreakLoop=off
  Series RLC Branch6 : spsSeriesRLCBranchLib/Series RLC Branch  LConnTagsString=__new0  RConnTagsString=__new0  BranchType=R  Resistance=2  Inductance=4e-3  SetiL0=off  InitialCurrent=0  Capacitance=1e-6  Setx0=off  InitialVoltage=0  Measurements=None
  In : PMIOPort  Side=Left
  Out : PMIOPort  Port=2  Side=Right
  connections:
  Out/RConn1 -- Series RLC Branch6/RConn1 -- Breaker1/RConn1
  In/RConn1 -- Series RLC Branch6/LConn1 -- Breaker1/LConn1

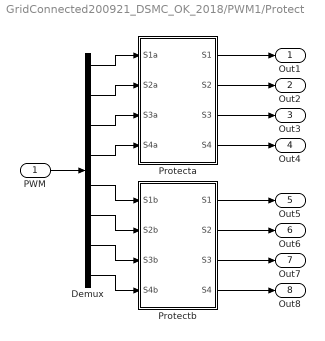
== system GridConnected200921_DSMC_OK_2018/PWM1/Protect ==
  PWM : Inport
  Demux : Demux  Outputs=8
  Protecta : Subsystem
  Protectb : Subsystem
  Out1 : Outport  VectorParamsAs1DForOutWhenUnconnected=off
  Out2 : Outport  Port=2  VectorParamsAs1DForOutWhenUnconnected=off
  Out3 : Outport  Port=3  VectorParamsAs1DForOutWhenUnconnected=off
  Out4 : Outport  Port=4  VectorParamsAs1DForOutWhenUnconnected=off
  Out5 : Outport  Port=5  VectorParamsAs1DForOutWhenUnconnected=off
  Out6 : Outport  Port=6  VectorParamsAs1DForOutWhenUnconnected=off
  Out7 : Outport  Port=7  VectorParamsAs1DForOutWhenUnconnected=off
  Out8 : Outport  Port=8  VectorParamsAs1DForOutWhenUnconnected=off
  wires:
  Protectb/2(S2) -> Out6/1
  Demux/3 -> Protecta/3(S3a)
  Demux/4 -> Protecta/4(S4a)
  Demux/2 -> Protecta/2(S2a)
  Protectb/3(S3) -> Out7/1
  Protectb/4(S4) -> Out8/1
  Demux/1 -> Protecta/1(S1a)
  Protectb/1(S1) -> Out5/1
  Protecta/4(S4) -> Out4/1
  Protecta/3(S3) -> Out3/1
  Protecta/2(S2) -> Out2/1
  Protecta/1(S1) -> Out1/1
  Demux/5 -> Protectb/1(S1b)
  Demux/6 -> Protectb/2(S2b)
  Demux/7 -> Protectb/3(S3b)
  Demux/8 -> Protectb/4(S4b)
  PWM/1 -> Demux/1

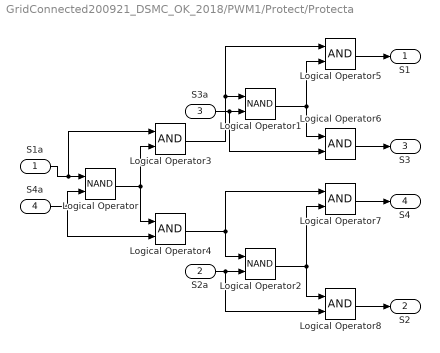
== system GridConnected200921_DSMC_OK_2018/PWM1/Protect/Protecta ==
  S1a : Inport
  S2a : Inport  Port=2
  S3a : Inport  Port=3
  S4a : Inport  Port=4
  Logical Operator : Logic  Operator=NAND  AllPortsSameDT=off  OutDataTypeStr=boolean
  Logical Operator1 : Logic  Operator=NAND  AllPortsSameDT=off  OutDataTypeStr=boolean
  Logical Operator2 : Logic  Operator=NAND  AllPortsSameDT=off  OutDataTypeStr=boolean
  Logical Operator{3..8} (6 alike) : Logic  AllPortsSameDT=off  OutDataTypeStr=boolean
  S1 : Outport  VectorParamsAs1DForOutWhenUnconnected=off
  S2 : Outport  Port=2  VectorParamsAs1DForOutWhenUnconnected=off
  S3 : Outport  Port=3  VectorParamsAs1DForOutWhenUnconnected=off
  S4 : Outport  Port=4  VectorParamsAs1DForOutWhenUnconnected=off
  wires:
  Logical Operator5/1 -> S1/1
  Logical Operator7/1 -> S4/1
  Logical Operator8/1 -> S2/1
  Logical Operator/1 -> Logical Operator4/1, Logical Operator3/2
  Logical Operator6/1 -> S3/1
  Logical Operator4/1 -> Logical Operator7/1, Logical Operator2/1
  Logical Operator1/1 -> Logical Operator5/2, Logical Operator6/1
  Logical Operator3/1 -> Logical Operator5/1, Logical Operator1/1
  Logical Operator2/1 -> Logical Operator7/2, Logical Operator8/1
  S1a/1 -> Logical Operator3/1, Logical Operator/1
  S4a/1 -> Logical Operator4/2, Logical Operator/2
  S3a/1 -> Logical Operator6/2, Logical Operator1/2
  S2a/1 -> Logical Operator8/2, Logical Operator2/2

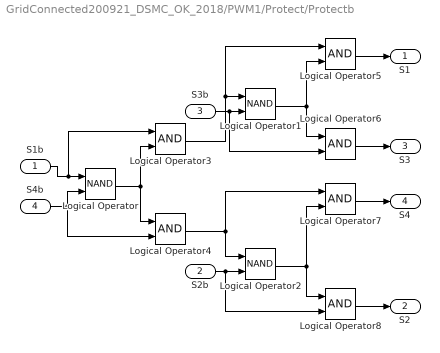
== system GridConnected200921_DSMC_OK_2018/PWM1/Protect/Protectb ==
  S1b : Inport
  S2b : Inport  Port=2
  S3b : Inport  Port=3
  S4b : Inport  Port=4
  Logical Operator : Logic  Operator=NAND  AllPortsSameDT=off  OutDataTypeStr=boolean
  Logical Operator1 : Logic  Operator=NAND  AllPortsSameDT=off  OutDataTypeStr=boolean
  Logical Operator2 : Logic  Operator=NAND  AllPortsSameDT=off  OutDataTypeStr=boolean
  Logical Operator{3..8} (6 alike) : Logic  AllPortsSameDT=off  OutDataTypeStr=boolean
  S1 : Outport  VectorParamsAs1DForOutWhenUnconnected=off
  S2 : Outport  Port=2  VectorParamsAs1DForOutWhenUnconnected=off
  S3 : Outport  Port=3  VectorParamsAs1DForOutWhenUnconnected=off
  S4 : Outport  Port=4  VectorParamsAs1DForOutWhenUnconnected=off
  wires:
  S2b/1 -> Logical Operator2/2, Logical Operator8/2
  S3b/1 -> Logical Operator1/2, Logical Operator6/2
  S4b/1 -> Logical Operator/2, Logical Operator4/2
  S1b/1 -> Logical Operator/1, Logical Operator3/1
  Logical Operator2/1 -> Logical Operator8/1, Logical Operator7/2
  Logical Operator3/1 -> Logical Operator1/1, Logical Operator5/1
  Logical Operator1/1 -> Logical Operator6/1, Logical Operator5/2
  Logical Operator4/1 -> Logical Operator2/1, Logical Operator7/1
  Logical Operator6/1 -> S3/1
  Logical Operator/1 -> Logical Operator3/2, Logical Operator4/1
  Logical Operator8/1 -> S2/1
  Logical Operator7/1 -> S4/1
  Logical Operator5/1 -> S1/1

== matlab function GridConnected200921_DSMC_OK_2018/PWM1/Switch_Uc ==
  data: I input; uc1 input; uc2 input; Uc1 output; Uc2 output
function [Uc1,Uc2] = Switch(I,uc1,uc2)
%#codegen
%a
Uc1 = 0;
Uc2 = 0;
if I < 0
    Uc1 = uc1;
    Uc2 = uc2;
end
if I >= 0
    Uc1 = uc2;
    Uc2 = uc1;
end
end

== matlab function GridConnected200921_DSMC_OK_2018/PWM1/Duty_Balance_Cap ==
  data: u input; d1a output; d4a output; d1b output; d4b output; uc1 input; uc2 input
function [d1a,d4a,d1b,d4b] = Duty(u,uc1,uc2)
%#codegen
%a
if (uc1 <= uc2) 
    d1a = u - 1;
else 
    d1a = u;
end
if (uc1 >= uc2);
    d4a = u + 2;
else 
    d4a = u + 1;
end

%b
if (uc1 >= uc2);
    d1b = u + 1;
else
    d1b = u + 2;
end
if (uc1 <= uc2) 
    d4b = u;
else
    d4b = u - 1;
end
end
